simulink model "f16"  (R2022a)
settings: Solver=VariableStepAuto  StartTime=0.0  StopTime=inf  RelTol=1e-3
undefined symbols (not defined in the file or in its folder): Receive, Send
libraries: aerolibfltsims x2, rllib x1
settings Model: Creator=sherwin kumar  LastModifiedBy=sherwin kumar

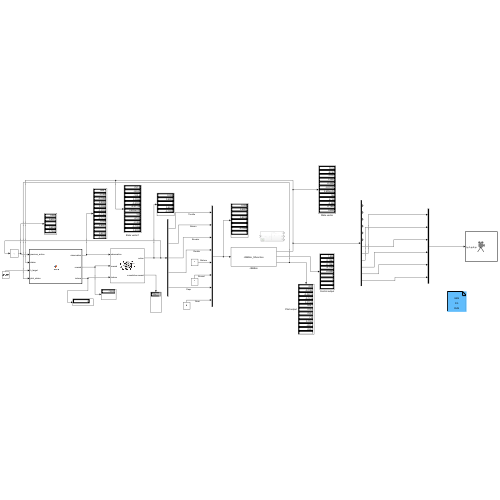
[thumbnail: Simulink's stored preview of the top-level diagram]
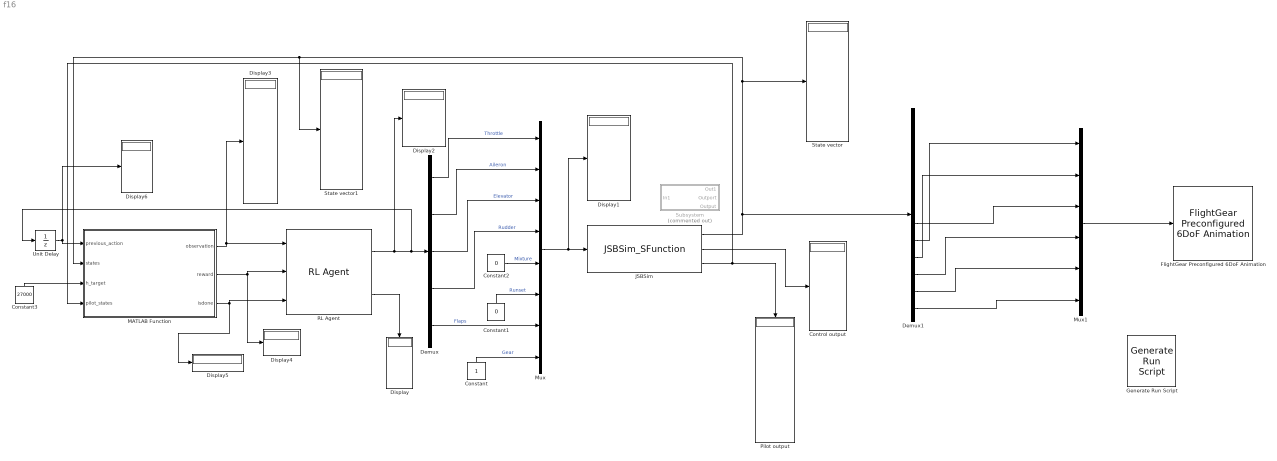
== system f16 ==
  Constant : Constant
  Constant1 : Constant  Value=0
  Constant2 : Constant  Value=0
  Constant3 : Constant  Value=27000
  Control output : Display
  Demux : Demux  Outputs=5
  Demux1 : Demux  Outputs=12
  Display{,1..6} (7 alike) : Display
  FlightGear Preconfigured 6DoF Animation : aerolibfltsims/FlightGear Preconfigured 6DoF Animation  xFlightGearVersion=v2019.1  DestinationIpAddress=127.0.0.1  DestinationPort=5502  SampleTime=1/30  packetVersion=24
  Generate Run Script : aerolibfltsims/Generate Run Script  Architecture=Default  dataFlow=Send-Receive  GeometryModelName=f16  AirportId=KSFO  RunwayId=10L  InitialAltitude=30000  InitialHeading=0  OffsetDistance=0  OffsetAzimuth=0  InstallScenery=off  DisableShaders=on  OriginAddress=127.0.0.1  DestinationPort=5502  OriginPort=5505  LocalAddress=127.0.0.1  OutputFileName=runfg.bat  FlightGearBaseDirectory=C:\Program Files\FlightGear
  JSBSim : S-Function  FunctionName=JSBSim_SFunction  Parameters='f16', 0.0083333, 0, 'scripts/f16_test', 'f16_init', 'f16_io'  SFunctionDeploymentMode=off  EnableBusSupport=off
  MATLAB Function : MATLAB Function  TreatAsAtomicUnit=on
  Mux : Mux  Inputs=8
  Mux1 : Mux  Inputs=6
  Pilot output : Display
  RL Agent : rllib/RL Agent  Agent=modelTraining  ExternalActionAsInput=off  ProvideLastAction=off  ProvideCumRwd=on  TreatAsDirectFeedthrough=on  UseStrictObservationDataTypes=off
  State vector : Display
  State vector1 : Display
  Subsystem : Subsystem  Commented=on
  Unit Delay : UnitDelay  SampleTime=-1  HasFrameUpgradeWarning=on
  wires:
  MATLAB Function/1(observation) -> RL Agent/1, Display3/1
  MATLAB Function/2(reward) -> RL Agent/2, Display4/1
  RL Agent/1 -> Display2/1, Unit Delay/1, Demux/1
  Demux/1 -> Mux/1  "Throttle"
  Demux/2 -> Mux/2  "Aileron"
  Demux/3 -> Mux/3  "Elevator"
  Demux/4 -> Mux/4  "Rudder"
  Demux/5 -> Mux/7  "Flaps"
  Constant/1 -> Mux/8  "Gear"
  Constant1/1 -> Mux/6  "Runset"
  Constant2/1 -> Mux/5  "Mixture"
  Mux/1 -> Display1/1, JSBSim/1
  Unit Delay/1 -> Display6/1, MATLAB Function/1(previous_action)
  Constant3/1 -> MATLAB Function/3(h_target)
  MATLAB Function/3(isdone) -> RL Agent/3, Display5/1
  RL Agent/2 -> Display/1
  JSBSim/2 -> Control output/1
  JSBSim/3 -> MATLAB Function/4(pilot_states), Pilot output/1
  JSBSim/1 -> State vector/1, State vector1/1, MATLAB Function/2(states), Demux1/1
  Mux1/1 -> FlightGear Preconfigured 6DoF Animation/1
  Demux1/7 -> Mux1/3
  Demux1/10 -> Mux1/4
  Demux1/11 -> Mux1/5
  Demux1/12 -> Mux1/6
  Demux1/8 -> Mux1/1
  Demux1/9 -> Mux1/2

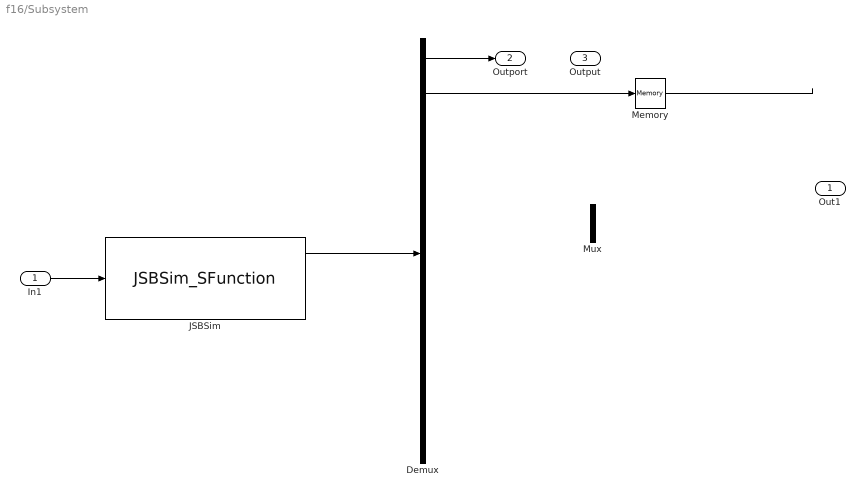
== system f16/Subsystem ==
  In1 : Inport
  Demux : Demux  Outputs=12
  JSBSim : S-Function  FunctionName=JSBSim_SFunction  Parameters='f16', 0.0083333, 0, 'scripts/f16_test', 'f16_init', 'f16_io'  SFunctionDeploymentMode=off  EnableBusSupport=off
  Memory : Memory
  Mux : Mux  Inputs=2
  Out1 : Outport
  Outport : Outport  Port=2
  Output : Outport  Port=3
  wires:
  In1/1 -> JSBSim/1
  JSBSim/1 -> Demux/1
  Demux/1 -> Outport/1
  Demux/2 -> Memory/1
  Memory/1 -> ?

== matlab function f16/MATLAB Function ==
  data: previous_action input; observation output; states input; h_target input; pilot_states input; reward output; isdone output

function [observation, reward, isdone] = Reward(previous_action, states, h_target, pilot_states)
     
    h = h_target - states(7);%dont get it
    %fprintf(states);
    phi = states(10);
    %fprintf(psi);
    p = states(4);
    %fprintf(p);
    q = states(5);
    %fprintf(q);
    alpha = pilot_states(2);
    beta = pilot_states(4);
    throttle_cmd = previous_action(1);
    roll_cmd = previous_action(2);
    pitch_cmd = previous_action(3);
    yaw_cmd = previous_action(4);
    flap_cmd = previous_action(5);
    if states(11)>180
        theta = -(2*180 - states(11));
    else
        %fprintf(phi);
        theta = states(11);
    end
    if states(12)>180
        psi = -(2*180 - states(12));
    else
        psi = states(12);
    end
    
    %Rewards
    h_reward = hyperbolicPenalty(h, -5, 5, 1/398, 0);
    roll_reward = hyperbolicPenalty(phi, -0.02, 0.02, 125/78, 0);
    pitch_reward = hyperbolicPenalty(theta, -0.02, 0.02, 125/78, 0);
    heading_reward = hyperbolicPenalty(psi, -0.02, 0.02, 125/78, 0);
    roll_rate_reward = hyperbolicPenalty(p, -0.1, 0.1, 125/78, 0);
    pitch_rate_reward = hyperbolicPenalty(q, -0.1, 0.1, 125/78, 0);
    %disp("Rewards:");
    
    if abs(h)>3000
        reward = -1000;
        isdone=0;
    else
        reward = -(h_reward + roll_reward + pitch_reward + heading_reward + roll_rate_reward + pitch_rate_reward);
        isdone = 0;
    end
    observation = [h, phi, theta, psi, p, q, alpha, beta, throttle_cmd, roll_cmd, pitch_cmd, yaw_cmd, flap_cmd];
end
